simulink model "IEEE_30_Bus_System"  (R2021a)
settings: Solver=FixedStepDiscrete  StartTime=0.0  StopTime=0.5  FixedStep=50e-6  RelTol=1e-3
undefined symbols (not defined in the file): Angle, Magnitude, V_890, Vnom1
libraries: spsThreePhasePISectionLineLib x37, spsThreePhaseVIMeasurementLib x30, spsLoadFlowBusLib x30, spsThreePhaseSeriesRLCLoadLib x21, spsThreePhaseSourceLib x6, spsThreePhaseTransformerTwoWindingsLib x4, spspowerguiLib x1
(part 2 of 2)

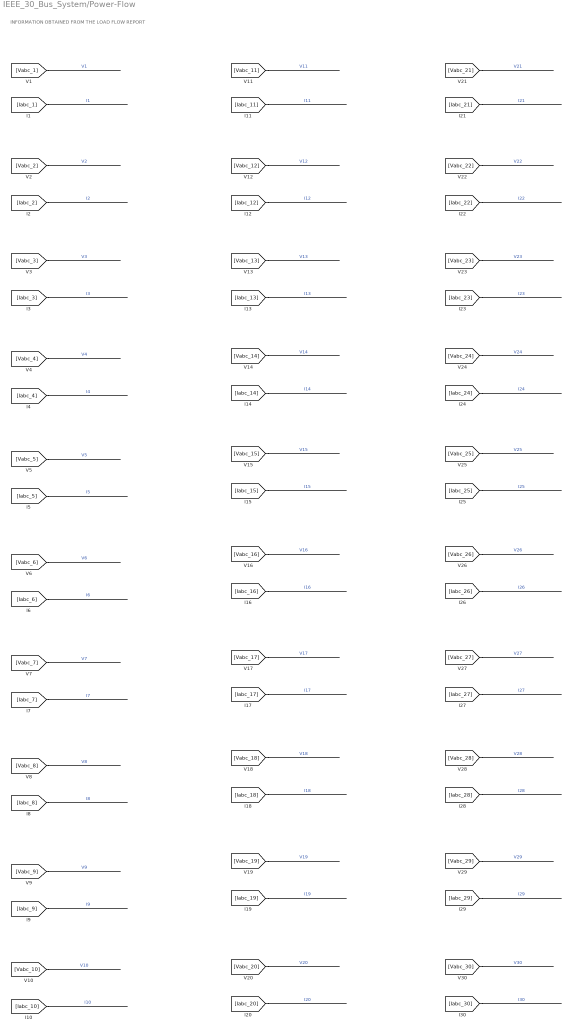
== system IEEE_30_Bus_System/Power-Flow ==
  note: INFORMATION OBTAINED FROM THE LOAD FLOW REPORT
  wires:
  [Vabc_1] -> ?  "V1"
  [Iabc_1] -> ?  "I1"
  [Vabc_2] -> ?  "V2"
  [Iabc_2] -> ?  "I2"
  [Iabc_3] -> ?  "I3"
  [Vabc_3] -> ?  "V3"
  [Vabc_4] -> ?  "V4"
  [Iabc_4] -> ?  "I4"
  [Vabc_5] -> ?  "V5"
  [Iabc_5] -> ?  "I5"
  [Vabc_6] -> ?  "V6"
  [Iabc_6] -> ?  "I6"
  [Vabc_7] -> ?  "V7"
  [Iabc_7] -> ?  "I7"
  [Vabc_8] -> ?  "V8"
  [Iabc_8] -> ?  "I8"
  [Vabc_9] -> ?  "V9"
  [Iabc_9] -> ?  "I9"
  [Vabc_10] -> ?  "V10"
  [Iabc_10] -> ?  "I10"
  [Iabc_18] -> ?  "I18"
  [Vabc_18] -> ?  "V18"
  [Iabc_13] -> ?  "I13"
  [Vabc_13] -> ?  "V13"
  [Iabc_11] -> ?  "I11"
  [Vabc_16] -> ?  "V16"
  [Iabc_16] -> ?  "I16"
  [Iabc_17] -> ?  "I17"
  [Vabc_17] -> ?  "V17"
  [Vabc_11] -> ?  "V11"
  [Iabc_12] -> ?  "I12"
  [Vabc_20] -> ?  "V20"
  [Iabc_20] -> ?  "I20"
  [Vabc_12] -> ?  "V12"
  [Iabc_19] -> ?  "I19"
  [Iabc_15] -> ?  "I15"
  [Vabc_19] -> ?  "V19"
  [Vabc_15] -> ?  "V15"
  [Vabc_14] -> ?  "V14"
  [Iabc_14] -> ?  "I14"
  [Iabc_26] -> ?  "I26"
  [Vabc_27] -> ?  "V27"
  [Vabc_26] -> ?  "V26"
  [Iabc_21] -> ?  "I21"
  [Vabc_23] -> ?  "V23"
  [Vabc_28] -> ?  "V28"
  [Iabc_27] -> ?  "I27"
  [Iabc_28] -> ?  "I28"
  [Vabc_24] -> ?  "V24"
  [Vabc_25] -> ?  "V25"
  [Iabc_23] -> ?  "I23"
  [Vabc_29] -> ?  "V29"
  [Iabc_24] -> ?  "I24"
  [Iabc_25] -> ?  "I25"
  [Vabc_30] -> ?  "V30"
  [Vabc_22] -> ?  "V22"
  [Iabc_29] -> ?  "I29"
  [Iabc_22] -> ?  "I22"
  [Iabc_30] -> ?  "I30"
  [Vabc_21] -> ?  "V21"
